simulink model "CH4_3C4"  (Simulink 7.5)
settings: Solver=ode45  StartTime=0.0  StopTime=3  RelTol=1e-3
undefined symbols (not defined in the file or in its folder): Fs, sided, Two
libraries: dspsnks4 x1
settings Model: Creator=my2  LastModifiedBy=xnote
settings DebuggingCC: FcnCallInpInsideContextMsg=Enable All  StateNameClashWarn=none
settings CodeAppCC: CustomSymbolStrType=$N$R$M_T
settings GRTTargetCC: TargetFunctionLibrary=C89/C90 (ANSI)

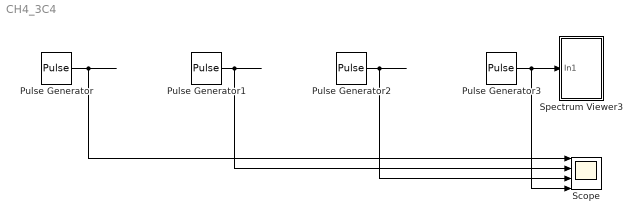
== system CH4_3C4 ==
  Pulse Generator{,1..3} (4 alike) : DiscretePulseGenerator  PulseType=Time based  Amplitude=1  Period=10  PulseWidth=5  PhaseDelay=0  SampleTime=1
  Scope : Scope  NumInputPorts=4
      settings: TimeRange=0.002  YMin=-0.5~-0.5~-0.5~-0.5  YMax=2~2~2~2  DataFormat=Array
  Spectrum Viewer3 : Subsystem
  wires:
  Pulse Generator/1 -> Scope/1
  Pulse Generator1/1 -> Scope/2
  Pulse Generator2/1 -> Scope/3
  Pulse Generator3/1 -> Spectrum Viewer3/1(In1), Scope/4

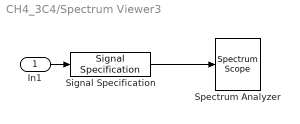
== system CH4_3C4/Spectrum Viewer3 ==
  In1 : Inport
  Signal Specification : SignalSpecification  SampleTime=1/32e4
  Spectrum Analyzer : dspsnks4/Spectrum Scope  DialogController=dspdialog.SpectrumScope  DialogControllerArgs=DataTag0  SystemSampleTime=-1  ScopeProperties=on  Domain=Frequency  HorizSpan=1  UseBuffer=on  BufferSize=1024  Overlap=64  inpFftLenInherit=on  FFTlength=1024  numAvg=200  DisplayProperties=off  AxisGrid=on  Memory=off  FrameNumber=on  AxisLegend=off  AxisZoom=off  OpenScopeAtSimStart=on  OpenScopeImmediately=off  FigPos="[8  291  752  208]"  AxisProperties=off  XUnits=Hertz  XRange=Two-sided ((-Fs/2...Fs/2])  XDisplay=0  InheritXIncr=on  XIncr=1.0  XLabel=Samples  XLimit=Auto  YUnits=Watts/Hertz  XMax=1  XMin=0  YLabel=Magnitude-squared, dB  LineProperties=off  wintypeSpecScope=Hann  RsSpecScope=50  betaSpecScope=5  winsampSpecScope=Symmetric  XAxisParamsVer=6.8
      settings: YMin=-6.1035e-009  YMax=3.4932e-005
  wires:
  In1/1 -> Signal Specification/1
  Signal Specification/1 -> Spectrum Analyzer/1
